simulink model "FonctionBFenZ"  (R2020a)
settings: Solver=VariableStepAuto  StartTime=0.0  StopTime=0.04  RelTol=1e-3
values from neighbouring files (symbols this model uses):
  denF = [t1*t2 t1+t2 1]    [correcteur2.m]
  denG = [Rmoteur*t_elec Rmoteur]    [correcteur2.m]
  numF = [Kretour]    [correcteur2.m]
  numG = [2*E]    [correcteur2.m]
  Te = 1/Fe    (= 0.000277777777778)    [correcteur.m]    (also in correcteur2.m)
libraries: cstblocks x1
settings Model: Creator=predon  LastModifiedBy=predon

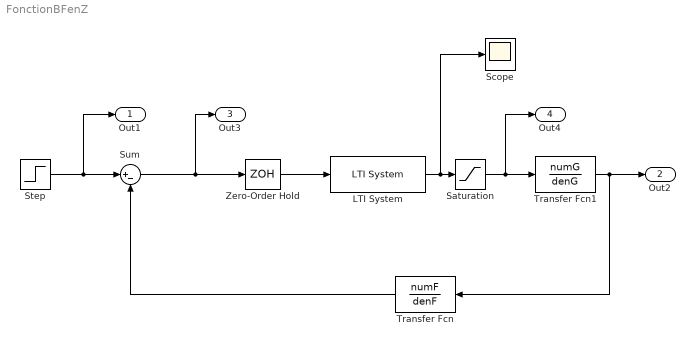
== system FonctionBFenZ ==
  LTI System : cstblocks/LTI System  sys=Cz  IC=[]
  Saturation : Saturate
  Scope : Scope
  Step : Step  Time=0.02  After=0.5  SampleTime=0
  Sum : Sum  Inputs=|+-
  Transfer Fcn : TransferFcn  Numerator=numF  Denominator=denF
  Transfer Fcn1 : TransferFcn  Numerator=numG  Denominator=denG
  Zero-Order Hold : ZeroOrderHold  SampleTime=Te
  Out1 : Outport  SignalName=Icons
  Out2 : Outport  Port=2  SignalName=Is
  Out3 : Outport  Port=3  SignalName=Erreur
  Out4 : Outport  Port=4  SignalName=Alpha
  wires:
  Transfer Fcn1/1 -> Out2/1, Transfer Fcn/1
  Step/1 -> Out1/1, Sum/1
  Sum/1 -> Zero-Order Hold/1, Out3/1
  Transfer Fcn/1 -> Sum/2
  LTI System/1 -> Scope/1, Saturation/1
  Saturation/1 -> Transfer Fcn1/1, Out4/1
  Zero-Order Hold/1 -> LTI System/1
